simulink model "training"  (R2025a)
settings: Solver=VariableStepAuto  StartTime=0.0  StopTime=1000  RelTol=1e-3
undefined symbols (not defined in the file or in its folder): dspblkCoreblockFVToolHelper, gcbh, teacherTaps
settings Model: Creator=Mayur  LastModifiedBy=Mayur

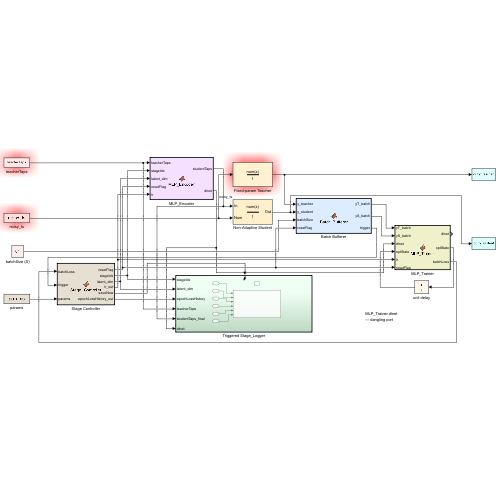
[thumbnail: Simulink's stored preview of the top-level diagram]
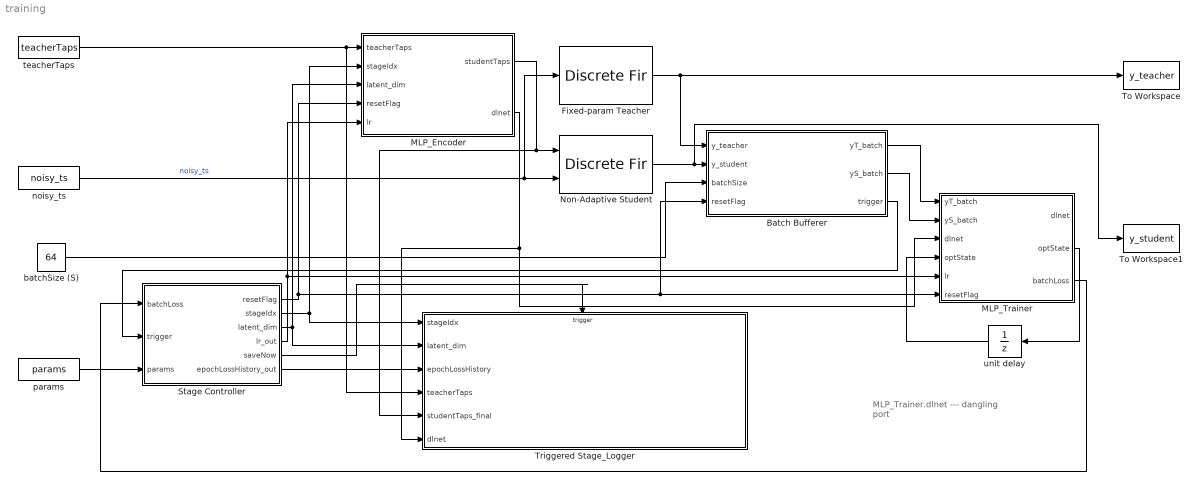
== system training ==
  note: MLP_Trainer.dlnet
      | --- dangling port
  Batch Bufferer : MATLAB Function  TreatAsAtomicUnit=on
  Fixed-param Teacher : DiscreteFir  LoadFcn=dspblkCoreblockFVToolHelper(gcbh,'load');  Coefficients=teacherTaps(:)'
      settings: CopyFcn=dspblkCoreblockFVToolHelper(gcbh,'copy');  DeleteFcn=dspblkCoreblockFVToolHelper(gcbh,'close');  ModelCloseFcn=dspblkCoreblockFVToolHelper(gcbh,'close');  PreSaveFcn=dspblkCoreblockFVToolHelper(gcbh,'presave');  PostSaveFcn=dspblkCoreblockFVToolHelper(gcbh,'postsave');  CloseFcn=dspblkCoreblockFVToolHelper(gcbh,'close');
  MLP_Encoder : MATLAB Function  TreatAsAtomicUnit=on
  MLP_Trainer : MATLAB Function  TreatAsAtomicUnit=on
  Non-Adaptive Student : DiscreteFir  LoadFcn=dspblkCoreblockFVToolHelper(gcbh,'load');  CoefSource=Input port
      settings: CopyFcn=dspblkCoreblockFVToolHelper(gcbh,'copy');  DeleteFcn=dspblkCoreblockFVToolHelper(gcbh,'close');  ModelCloseFcn=dspblkCoreblockFVToolHelper(gcbh,'close');  PreSaveFcn=dspblkCoreblockFVToolHelper(gcbh,'presave');  PostSaveFcn=dspblkCoreblockFVToolHelper(gcbh,'postsave');  CloseFcn=dspblkCoreblockFVToolHelper(gcbh,'close');  InputPortMap=u0,u1
  Stage Controller : MATLAB Function  TreatAsAtomicUnit=on
  To Workspace : ToWorkspace  VariableName=y_teacher  SaveFormat=Timeseries  SampleTime=-1
  To Workspace1 : ToWorkspace  VariableName=y_student  SaveFormat=Timeseries  SampleTime=-1
  Triggered Stage_Logger : Subsystem  TreatAsAtomicUnit=on
  batchSize (S) : Constant  Value=64
  noisy_ts : FromWorkspace  VariableName=noisy_ts  SampleTime=1
  params : FromWorkspace  VariableName=params
  teacherTaps : FromWorkspace  VariableName=teacherTaps
  unit delay : UnitDelay  SampleTime=-1  HasFrameUpgradeWarning=on
  wires:
  Stage Controller/1(resetFlag) -> MLP_Encoder/4(resetFlag), Batch Bufferer/4(resetFlag), MLP_Trainer/6(resetFlag)
  teacherTaps/1 -> Triggered Stage_Logger/4(teacherTaps), MLP_Encoder/1(teacherTaps)
  Stage Controller/3(latent_dim) -> Triggered Stage_Logger/2(latent_dim), MLP_Encoder/3(latent_dim)
  Stage Controller/2(stageIdx) -> Triggered Stage_Logger/1(stageIdx), MLP_Encoder/2(stageIdx)
  MLP_Encoder/1(studentTaps) -> Non-Adaptive Student/1, Triggered Stage_Logger/5(studentTaps_final)
  Stage Controller/4(lr_out) -> MLP_Trainer/5(lr), MLP_Encoder/5(lr)
  noisy_ts/1 -> Non-Adaptive Student/2, Fixed-param Teacher/1  "noisy_ts"
  Fixed-param Teacher/1 -> To Workspace/1, Batch Bufferer/1(y_teacher)
  batchSize (S)/1 -> Batch Bufferer/3(batchSize)
  Batch Bufferer/1(yT_batch) -> MLP_Trainer/1(yT_batch)
  Batch Bufferer/2(yS_batch) -> MLP_Trainer/2(yS_batch)
  Batch Bufferer/3(trigger) -> Stage Controller/2(trigger)
  MLP_Trainer/3(batchLoss) -> Stage Controller/1(batchLoss)
  MLP_Encoder/2(dlnet) -> Triggered Stage_Logger/6(dlnet), MLP_Trainer/3("dlnet ")
  MLP_Trainer/2(optState) -> unit delay/1
  unit delay/1 -> MLP_Trainer/4("optState ")
  params/1 -> Stage Controller/3(params)
  Stage Controller/6(epochLossHistory_out) -> Triggered Stage_Logger/3(epochLossHistory)
  Stage Controller/5(saveNow) -> Triggered Stage_Logger/Trigger
  Non-Adaptive Student/1 -> To Workspace1/1, Batch Bufferer/2(y_student)

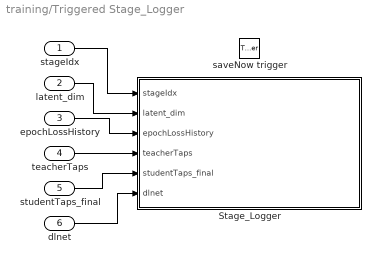
== system training/Triggered Stage_Logger ==
  stageIdx : Inport
  latent_dim : Inport  Port=2
  epochLossHistory : Inport  Port=3
  teacherTaps : Inport  Port=4
  studentTaps_final : Inport  Port=5
  dlnet : Inport  Port=6
  saveNow trigger : TriggerPort  VariantControl=(inherit)
  Stage_Logger : MATLAB Function  TreatAsAtomicUnit=on
  wires:
  stageIdx/1 -> Stage_Logger/1(stageIdx)
  latent_dim/1 -> Stage_Logger/2(latent_dim)
  epochLossHistory/1 -> Stage_Logger/3(epochLossHistory)
  teacherTaps/1 -> Stage_Logger/4(teacherTaps)
  studentTaps_final/1 -> Stage_Logger/5(studentTaps_final)
  dlnet/1 -> Stage_Logger/6(dlnet)

== matlab function training/Batch Bufferer ==
  data: y_teacher input; yT_batch output; y_student input; batchSize input; resetFlag input; yS_batch output; trigger output
function [yT_batch, yS_batch, trigger] = Batch_Bufferer(y_teacher, y_student, batchSize, resetFlag)
% Batch_Bufferer — Collects synchronized teacher/student batches
% --------------------------------------------------------------------
% Inputs:
%   y_teacher  : Current teacher output sample
%   y_student  : Current student output sample
%   batchSize  : Batch length for accumulation
%   resetFlag  : Reset buffer between clips/stages
%
% Outputs:
%   yT_batch   : Full teacher batch [feat × batchSize]
%   yS_batch   : Full student batch [feat × batchSize]
%   trigger    : Boolean flag when batch full
% --------------------------------------------------------------------

persistent bufferT bufferS count numFeatures

if isempty(bufferT) || resetFlag
    numFeatures = numel(y_teacher);
    bufferT = zeros(numFeatures, batchSize, 'single');
    bufferS = zeros(numFeatures, batchSize, 'single');
    count = 0;
    trigger = false;
    yT_batch = zeros(numFeatures, batchSize, 'single');
    yS_batch = zeros(numFeatures, batchSize, 'single');

    if resetFlag    % stage reset case -------------------
        fprintf('[Batch_Bufferer] Buffer reset (new stage).\n');
    end

    return;
end

% =====================================================
% Step 1 — Accumulate current samples
% =====================================================
count = count + 1;
bufferT(:, count) = single(y_teacher(:));
bufferS(:, count) = single(y_student(:));

% =====================================================
% Step 2 — Check if batch full
% =====================================================
if count >= batchSize
    yT_batch = bufferT;
    yS_batch = bufferS;
    trigger = true;

    % Reset for next batch
    bufferT(:) = 0;
    bufferS(:) = 0;
    count = 0;
else
    yT_batch = zeros(numFeatures, batchSize, 'single');
    yS_batch = zeros(numFeatures, batchSize, 'single');
    trigger = false;
end

end

== matlab function training/MLP_Encoder ==
  data: teacherTaps input; studentTaps output; stageIdx input; latent_dim input; resetFlag input; lr input; dlnet output
function [studentTaps, dlnet] = MLP_Encoder(teacherTaps, stageIdx, latent_dim, resetFlag, lr)
%#codegen
persistent dlnet_prev stageIdx_prev

% ========================
% 1. Initialize / Expand
% ========================
if isempty(dlnet_prev) || resetFlag || stageIdx ~= stageIdx_prev
    fprintf('Initializing/Expanding MLP for Stage %d...\n', stageIdx);

    if isempty(dlnet_prev)
        % ---- Stage 1: create base network ----
        layers = [
            featureInputLayer(length(teacherTaps), 'Name', 'input')
            fullyConnectedLayer(64, 'Name', 'fc1')
            reluLayer('Name', 'relu1')
            fullyConnectedLayer(latent_dim, 'Name', 'latent_stage1')
        ];
        lgraph = layerGraph(layers);
        dlnet_prev = dlnetwork(lgraph);

    else
        % ---- Later stage: transform + expand ----
        netLayers = layerGraph(dlnet_prev);

        % Step 1: Get last latent layer name
        prevLatentName = sprintf('latent_stage%d', stageIdx_prev);

        % Step 2: Rename old latent layer to FC_hidden_stageN
        newHiddenName = sprintf('fc_hidden_stage%d', stageIdx_prev);
        netLayers = replaceLayer(netLayers, prevLatentName, ...
            fullyConnectedLayer(latent_dim, 'Name', newHiddenName));

        % Step 3: Add ReLU + new Latent layer
        reluName = sprintf('relu_stage%d', stageIdx);
        newLatentName = sprintf('latent_stage%d', stageIdx);

        newLayers = [
            reluLayer('Name', reluName)
            fullyConnectedLayer(latent_dim, 'Name', newLatentName)
        ];

        % Step 4: Connect old hidden → ReLU
        netLayers = addLayers(netLayers, newLayers);
        netLayers = connectLayers(netLayers, newHiddenName, reluName);

        % Step 5: Build new dlnetwork
        dlnet_prev = dlnetwork(netLayers);
    end

    stageIdx_prev = stageIdx;
end

% ========================
% 2. Forward Pass
% ========================
dlX = dlarray(single(teacherTaps(:)), "CB"); % column batch
dlY = forward(dlnet_prev, dlX);

studentTaps = extractdata(dlY);
studentTaps = studentTaps(:)';

% ========================
% 3. Return
% ========================
dlnet = dlnet_prev;

end

== matlab function training/Stage Controller ==
  data: batchLoss input; resetFlag output; trigger input; params input; stageIdx output; latent_dim output; lr_out output; saveNow output; epochLossHistory_out output
function [resetFlag, stageIdx, latent_dim, lr_out, saveNow, epochLossHistory_out] = Stage_Controller(batchLoss, trigger, params)
% Stage_Controller — governs stage transitions and convergence
% --------------------------------------------------------------

persistent epoch batchCount epochLossAccum epochLossHistory ...
           noImproveCount prevMovingAvg stageIdxPrev lrPrev

% =====================================================
% Initialization
% =====================================================
if isempty(stageIdxPrev)
    stageIdxPrev = 1;
    epoch = 0;
    batchCount = 0;
    epochLossAccum = [];
    epochLossHistory = [];
    noImproveCount = 0;
    prevMovingAvg = inf;
    lrPrev = params.lr;
end

resetFlag = false;
saveNow   = false;
epochLossHistory_out = []; % ensure always defined

stageIdx   = stageIdxPrev;
latent_dim = params.student_latent_list(stageIdxPrev);
lr_out     = lrPrev;

% =====================================================
% Step 1 — Accumulate batch losses per epoch
% =====================================================
if trigger
    batchCount = batchCount + 1;
    epochLossAccum(end+1) = batchLoss;

    if batchCount >= params.B
        % -------------------------------
        % End of epoch reached
        % -------------------------------
        epoch = epoch + 1;
        epochMeanLoss = mean(epochLossAccum);
        epochLossHistory(end+1) = epochMeanLoss;
        epochLossHistory_out = epochLossHistory;  % expose to logger

        % Compute moving average
        if numel(epochLossHistory) >= params.mv_window
            movingAvg = mean(epochLossHistory(end - params.mv_window + 1:end));
        else
            movingAvg = mean(epochLossHistory);
        end

        % Improvement check
        if (prevMovingAvg - movingAvg) > params.tol
            noImproveCount = 0;
        else
            noImproveCount = noImproveCount + 1;
        end
        prevMovingAvg = movingAvg;

        % Display live diagnostics
        fprintf('[Stage %d] Epoch %d | Loss = %.6f | MA = %.6f | Pat = %d/%d\n', ...
            stageIdx, epoch, epochMeanLoss, movingAvg, noImproveCount, params.patience);

        % Reset accumulators for next epoch
        batchCount = 0;
        epochLossAccum = [];

        % -------------------------------
        % Step 2 — Convergence Check
        % -------------------------------
        if (noImproveCount >= params.patience) || (epoch >= params.maxEpochsPerStage)
            saveNow = true;  % signal to save before switching
        end
    end
end

% =====================================================
% Step 3 — Stage Transition Logic
% =====================================================
if saveNow
    epochLossHistory_out = epochLossHistory;

    % Move to next stage
    if stageIdxPrev < numel(params.student_latent_list)
        stageIdxPrev = stageIdxPrev + 1;
        latent_dim = params.student_latent_list(stageIdxPrev);
        resetFlag = true;
        fprintf('\n=== Stage %d complete. Moving to Stage %d (latent_dim = %d) ===\n', ...
            stageIdxPrev - 1, stageIdxPrev, latent_dim);
    else
        % No more stages left
        resetFlag = false;
        fprintf('\n=== All stages complete. Training finished. ===\n');
    end

    % Reset per-stage variables
    epoch = 0;
    batchCount = 0;
    epochLossAccum = [];
    epochLossHistory = [];
    noImproveCount = 0;
    prevMovingAvg = inf;
    lrPrev = params.lr;  % could implement lr decay schedule here
end

end

== matlab function training/MLP_Trainer ==
  data: yT_batch input; dlnet output; yS_batch input; dlnet input; optState input; lr input; resetFlag input; optState output; batchLoss output
function [dlnet, optState, batchLoss] = MLP_Trainer(yT_batch, yS_batch, dlnet, optState, lr, resetFlag)
% MLP_Trainer — Online runtime training block (Simulink-ready)
% ------------------------------------------------------------
% Responsibilities:
%   1. Compute MSE loss between teacher and student filter outputs
%   2. Backpropagate through the MLP (auto-diff)
%   3. Apply Adam update using Deep Learning Toolbox
%
% Inputs:
%   yT_batch, yS_batch : Buffers (vectors) from Teacher and Student filters
%   dlnet              : dlnetwork from MLP_Encoder
%   optState           : Adam optimizer state (struct)
%   lr                 : Learning rate
%   resetFlag          : Reset signal per stage
%
% Outputs:
%   dlnet              : Updated dlnetwork
%   optState           : Updated optimizer state
%   batchLoss          : Scalar MSE loss for the current batch
% ------------------------------------------------------------

% =====================================================
% Step 0 — Reset optimizer state if needed
% =====================================================
if isempty(optState) || resetFlag
    optState = [];
    disp('[MLP_Trainer] Optimizer state reset.');
end

% =====================================================
% Step 1 — Convert batch to dlarray
% =====================================================
dlY_T = dlarray(single(yT_batch(:)), "CB");
dlY_S = dlarray(single(yS_batch(:)), "CB");

% =====================================================
% Step 2 — Define loss function handle for dlfeval
% =====================================================
lossFcn = @(dlnet, dlY_T, dlY_S) ...
    mean((forward(dlnet, dlY_T) - dlY_S).^2, 'all');

% =====================================================
% Step 3 — Evaluate loss and compute gradients
% =====================================================
[batchLoss, gradients] = dlfeval(@modelGradients, dlnet, dlY_T, dlY_S);

% =====================================================
% Step 4 — Update weights with Adam optimizer
% =====================================================
[dlnet, optState] = adamupdate(dlnet, gradients, optState, lr);

% =====================================================
% Step 5 — Display optional debug info
% =====================================================
fprintf('[MLP_Trainer] Batch Loss: %.6f\n', gather(extractdata(batchLoss)));

end

% =====================================================
% Local helper function for gradient computation
% =====================================================
function [loss, gradients] = modelGradients(dlnet, dlY_T, dlY_S)
    % Forward pass (student output)
    yPred = forward(dlnet, dlY_T);
    % Mean Squared Error
    loss = mean((yPred - dlY_S).^2, 'all');
    % Backpropagate
    gradients = dlgradient(loss, dlnet.Learnables);
end

== matlab function training/Triggered Stage_Logger/Stage_Logger ==
  data: stageIdx input; latent_dim input; epochLossHistory input; teacherTaps input; studentTaps_final input; dlnet input
function Stage_Logger(stageIdx, latent_dim, epochLossHistory, teacherTaps, studentTaps_final, dlnet)
% Stage_Logger — Minimal per-stage logger for MLP KD training
% -----------------------------------------------------------
% Triggered once per stage when saveNow = true
%
% Inputs:
%   stageIdx          : Current stage index
%   latent_dim        : Latent dimension (K)
%   epochLossHistory  : Mean MSE values per epoch (from Stage_Controller)
%   teacherTaps       : Reference filter coefficients
%   studentTaps_final : Final student filter taps for this stage
%   dlnet             : Trained MLP_Encoder network
%
% Outputs:
%   None — writes results to disk (metrics, models, taps, plots)
% -----------------------------------------------------------

% ==============================================================
% 1. Directory Setup
% ==============================================================
baseDir = sprintf("results/Stage_%02d_lat%d", stageIdx, latent_dim);
mkdir(fullfile(baseDir, "metrics"));
mkdir(fullfile(baseDir, "models"));
mkdir(fullfile(baseDir, "taps"));
mkdir(fullfile(baseDir, "plots"));

% ==============================================================
% 2. Save Model + Student Taps
% ==============================================================
save(fullfile(baseDir, "models", sprintf("mlp_stage_%02d.mat", stageIdx)), ...
     "dlnet", "-v7.3");
save(fullfile(baseDir, "taps", sprintf("studentTaps_mlp_stage_%02d.mat", stageIdx)), ...
     "studentTaps_final");

% ==============================================================
% 3. Save Training Metrics (Mean MSE per Epoch)
% ==============================================================
Epoch = (1:numel(epochLossHistory))';
MSE   = epochLossHistory(:);
T = table(Epoch, MSE);
writetable(T, fullfile(baseDir, "metrics", ...
    sprintf("train_history_stage_%02d.csv", stageIdx)));

% ==============================================================
% 4. Plot: Epoch Loss Curve (hi-res)
% ==============================================================
f1 = figure('Visible', 'off', 'Position', [100 100 600 400]);
plot(Epoch, MSE, 'b-', 'LineWidth', 1.6);
xlabel('Epoch');
ylabel('Mean MSE');
title(sprintf('Stage %d (latent=%d) — Training Loss', stageIdx, latent_dim));
grid on;
set(gca, 'FontSize', 11);
set(gcf, 'PaperUnits', 'inches', 'PaperPosition', [0 0 6 4]);
print(f1, fullfile(baseDir, "plots", ...
    sprintf("loss_curve_stage_%02d.png", stageIdx)), '-dpng', '-r600');
close(f1);

% ==============================================================
% 5. Plot: Frequency Response Comparison (hi-res)
% ==============================================================
f2 = figure('Visible', 'off', 'Position', [100 100 600 400]);
[H_T, w] = freqz(teacherTaps, 1, 512);
[H_S, ~] = freqz(studentTaps_final, 1, 512);
plot(w/pi, 20*log10(abs(H_T) + eps), 'k-', 'LineWidth', 1.5); hold on;
plot(w/pi, 20*log10(abs(H_S) + eps), 'r--', 'LineWidth', 1.3);
xlabel('Normalized Frequency (\times\pi rad/sample)');
ylabel('Magnitude (dB)');
legend('Teacher', 'Student', 'Location', 'best');
title(sprintf('Stage %d (latent=%d) — Frequency Response', stageIdx, latent_dim));
grid on;
set(gca, 'FontSize', 11);
set(gcf, 'PaperUnits', 'inches', 'PaperPosition', [0 0 6 4]);
print(f2, fullfile(baseDir, "plots", ...
    sprintf("fr_compare_stage_%02d.png", stageIdx)), '-dpng', '-r600');
close(f2);

% ==============================================================
% 6. Completion Message
% ==============================================================
fprintf('[Stage_Logger] Stage %d (latent=%d) logged successfully.\n', ...
    stageIdx, latent_dim);
end
